simulink model "main"  (R2013a)
settings: Solver=ode45  StartTime=0.0  StopTime=40  RelTol=1e-3
undefined symbols (not defined in the file): National_Instruments, PCI, pin
libraries: simulink x5, rtwinlib x3
settings Model: Creator=CC LAB  LastModifiedBy=CC Lab

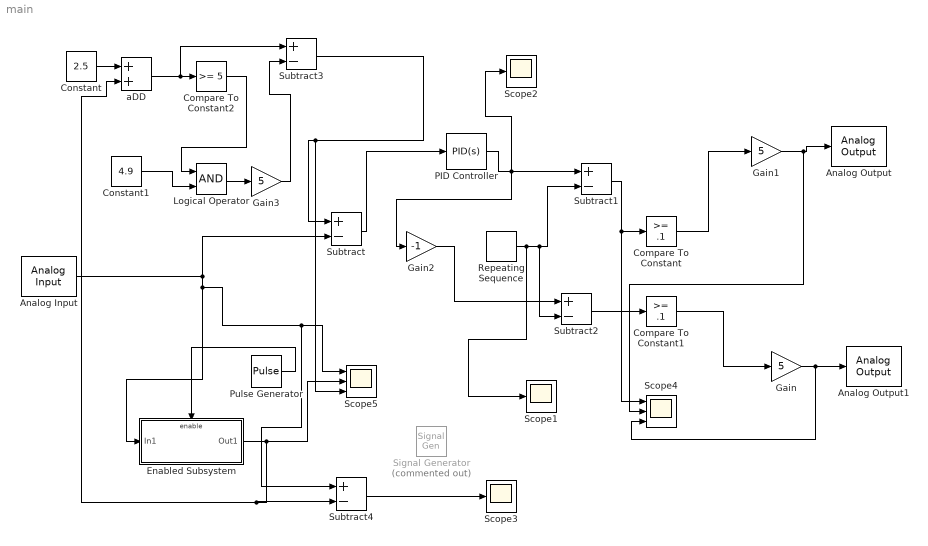
== system main ==
  Analog Input : rtwinlib/Analog Input  SampleTime=0.001  MaxMissedTicks=1000  ShowMissedTicks=off  YieldWhenWaiting=off  DrvName=National_Instruments/PCI-6221_37-pin  DrvAddress=0  DrvOptions=[0 0 0 0 0]  Channels=2  RangeMode=1  VoltRange=1  DataType=1
      settings: AttributesFormatString=National Instruments\nPCI-6221 37-pin [0h]
  Analog Output : rtwinlib/Analog Output  SampleTime=0.001  MaxMissedTicks=1000  ShowMissedTicks=off  YieldWhenWaiting=off  DrvName=National_Instruments/PCI-6221_37-pin  DrvAddress=0  DrvOptions=[0 0 0 0 0]  Channels=1  RangeMode=1  VoltRange=1  InitialValue=[]  FinalValue=0
      settings: AttributesFormatString=National Instruments\nPCI-6221 37-pin [0h]
  Analog Output1 : rtwinlib/Analog Output  SampleTime=0.001  MaxMissedTicks=1000  ShowMissedTicks=off  YieldWhenWaiting=off  DrvName=National_Instruments/PCI-6221_37-pin  DrvAddress=0  DrvOptions=[0 0 0 0 0]  Channels=2  RangeMode=1  VoltRange=1  InitialValue=[]  FinalValue=0
      settings: AttributesFormatString=National Instruments\nPCI-6221 37-pin [0h]
  Compare To Constant : simulink/Logic and Bit Operations/Compare To Constant  relop=>=  const=.1  OutDataTypeStr=uint8
  Compare To Constant1 : simulink/Logic and Bit Operations/Compare To Constant  relop=>=  const=.1  OutDataTypeStr=uint8
  Compare To Constant2 : simulink/Logic and Bit Operations/Compare To Constant  relop=>=  const=5  OutDataTypeStr=uint8
  Constant : Constant  Value=2.5
  Constant1 : Constant  Value=4.9
  Enabled Subsystem : Subsystem  TreatAsAtomicUnit=on
  Gain : Gain  Gain=5  OutDataTypeStr=double
  Gain1 : Gain  Gain=5  OutDataTypeStr=double
  Gain2 : Gain  Gain=-1
  Gain3 : Gain  Gain=5  OutDataTypeStr=double
  Logical Operator : Logic  AllPortsSameDT=off  OutDataTypeStr=boolean
  PID Controller : simulink/Continuous/PID Controller  Controller=PID  TimeDomain=Continuous-time  SampleTime=1  IntegratorMethod=Forward Euler  FilterMethod=Forward Euler  Form=Parallel  P=10  I=0.1  D=0  N=100  InitialConditionSource=internal  InitialConditionForIntegrator=0  InitialConditionForFilter=0  ExternalReset=none  LimitOutput=off  UpperSaturationLimit=inf  LowerSaturationLimit=-inf  LinearizeAsGain=on  AntiWindupMode=none  Kb=1  TrackingMode=off  Kt=1  PParamMin=[]  PParamMax=[]  IParamMin=[]  IParamMax=[]  DParamMin=[]  DParamMax=[]  NParamMin=[]  NParamMax=[]  KbParamMin=[]  KbParamMax=[]  KtParamMin=[]  KtParamMax=[]  POutMin=[]  POutMax=[]  IOutMin=[]  IOutMax=[]  DOutMin=[]  DOutMax=[]  NOutMin=[]  NOutMax=[]  KbOutMin=[]  KbOutMax=[]  KtOutMin=[]  KtOutMax=[]  IntegratorOutMin=[]  IntegratorOutMax=[]  FilterOutMin=[]  FilterOutMax=[]  SumOutMin=[]  SumOutMax=[]  SumI1OutMin=[]  SumI1OutMax=[]  SumI2OutMin=[]  SumI2OutMax=[]  SumI3OutMin=[]  SumI3OutMax=[]  SumDOutMin=[]  SumDOutMax=[]  SaturationOutMin=[]  SaturationOutMax=[]  IntegratorContinuousStateAttributes=''  IntegratorStateMustResolveToSignalObject=off  IntegratorRTWStateStorageClass=Auto  FilterContinuousStateAttributes=''  FilterStateMustResolveToSignalObject=off  FilterRTWStateStorageClass=Auto
  Pulse Generator : DiscretePulseGenerator  PulseType=Time based  Period=100  PulseWidth=0.1
  Repeating Sequence : simulink/Sources/Repeating Sequence  rep_seq_t=[0 .1]  rep_seq_y=[0 10]
  Scope1 : Scope
      settings: YMin=0  YMax=10
  Scope2 : Scope
      settings: YMin=-27.5  YMax=27.5  SaveName=ScopeData2
  Scope3 : Scope
      settings: YMin=1.925  YMax=2.5
  Scope4 : Scope  NumInputPorts=3
      settings: YMin=-40~0~0  YMax=30~5~5  SaveName=ScopeData4
  Scope5 : Scope  NumInputPorts=3
      settings: TimeRange=40  YMin=1.25~3.88481~1.38481  YMax=3.25~3.88481~1.38481  SaveName=ScopeData5
  Signal Generator : SignalGenerator  Commented=on  WaveForm=sawtooth  Amplitude=5  Frequency=100
  Subtract{,1..4} (5 alike) : Sum  Inputs=+-
  "aDD " : Sum
  wires:
  Subtract/1 -> PID Controller/1
  Analog Input/1 -> Enabled Subsystem/1(In1), Subtract4/1, Scope5/1, Subtract/2
  Compare To Constant/1 -> Gain1/1
  Compare To Constant1/1 -> Gain/1
  Gain/1 -> Scope4/3, Analog Output1/1
  PID Controller/1 -> Gain2/1, Subtract1/1, Scope2/1
  Subtract1/1 -> Scope4/1, Compare To Constant/1
  Subtract2/1 -> Compare To Constant1/1
  Gain2/1 -> Subtract2/1
  Gain1/1 -> Scope4/2, Analog Output/1
  Repeating Sequence/1 -> Scope1/1, Subtract2/2, Subtract1/2
  Pulse Generator/1 -> Enabled Subsystem/Enable
  Constant/1 -> "aDD "/1
  Enabled Subsystem/1(Out1) -> Subtract4/2, "aDD "/2, Scope5/2
  Compare To Constant2/1 -> Logical Operator/1
  Constant1/1 -> Logical Operator/2
  Logical Operator/1 -> Gain3/1
  "aDD "/1 -> Subtract3/1, Compare To Constant2/1
  Gain3/1 -> Subtract3/2
  Subtract3/1 -> Scope5/3, Subtract/1
  Subtract4/1 -> Scope3/1

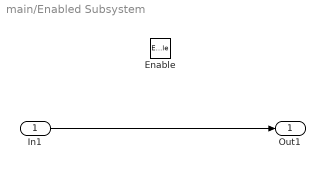
== system main/Enabled Subsystem ==
  In1 : Inport
  Enable : EnablePort
  Out1 : Outport
  wires:
  In1/1 -> Out1/1
